simulink model "engine"  (R2020b)
settings: Solver=VariableStepAuto  StartTime=0.0  StopTime=1  RelTol=1e-3
model workspace (MAT data in the model file):
  Tm = 6
  U_pr = 100
  k = 0.01
settings Model: Creator=anton  LastModifiedBy=anton

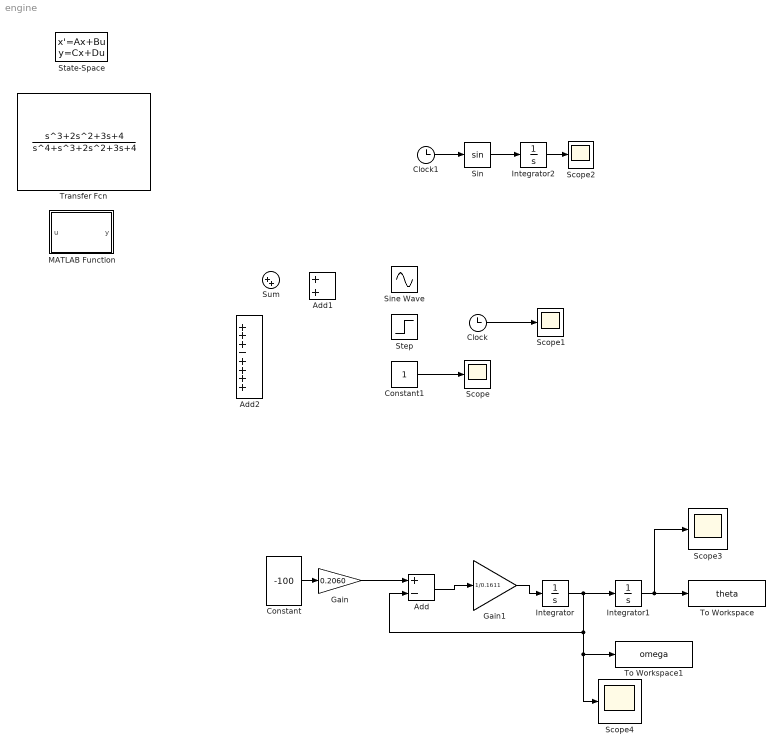
== system engine ==
  Add : Sum  Inputs=+-
  Add1 : Sum
  Add2 : Sum  Inputs=+++|-|++++
  Clock : Clock
  Clock1 : Clock
  Constant : Constant  Value=-100  SampleTime=-1
  Constant1 : Constant  SampleTime=-1
  Gain : Gain  Gain=0.2060
  Gain1 : Gain  Gain=1/0.1611
  Integrator : Integrator
  Integrator1 : Integrator
  Integrator2 : Integrator
  MATLAB Function : MATLAB Function  TreatAsAtomicUnit=on
  Scope{,1..4} (5 alike) : Scope
  Sin : Trigonometry
  Sine Wave : Sin  SampleTime=0
  State-Space : StateSpace  InitialCondition=0
  Step : Step  SampleTime=0
  Sum : Sum  Inputs=|++
  To Workspace : ToWorkspace  VariableName=theta  SaveFormat=Timeseries  SampleTime=-1
  To Workspace1 : ToWorkspace  VariableName=omega  SaveFormat=Timeseries  SampleTime=-1
  Transfer Fcn : TransferFcn  Numerator=[1 2 3 4]  Denominator=[1 1 2 3 4]
  wires:
  Constant/1 -> Gain/1
  Gain/1 -> Add/1
  Add/1 -> Gain1/1
  Gain1/1 -> Integrator/1
  Integrator/1 -> Scope4/1, To Workspace1/1, Add/2, Integrator1/1
  Constant1/1 -> Scope/1
  Clock/1 -> Scope1/1
  Clock1/1 -> Sin/1
  Sin/1 -> Integrator2/1
  Integrator2/1 -> Scope2/1
  Integrator1/1 -> Scope3/1, To Workspace/1

== matlab function engine/MATLAB Function ==
  data: u input; y output
function y = fcn(u)

y = u;
